simulink model "PreCondition"  (R2018b)
settings: Solver=FixedStepDiscrete  StartTime=0.0  StopTime=10.0  FixedStep=0.01  RelTol=1e-3
undefined symbols (not defined in the file or in its folder): EnergyMgLdShdRq1, HMI_2L_StMd10_Config_Val, HMI_2L_StMd11_Config_Val, HMI_2L_StMd12_Config_Val, HMI_2L_StMd13_Config_Val, HMI_2L_StMd14_Config_Val, HMI_2L_StMd15_Config_Val, HMI_2L_StMd16_Config_Val, HMI_2L_StMd17_Config_Val, HMI_2L_StMd18_Config_Val, HMI_2L_StMd19_Config_Val, HMI_2L_StMd1_Config_Val, HMI_2L_StMd20_Config_Val, HMI_2L_StMd21_Config_Val, HMI_2L_StMd22_Config_Val, HMI_2L_StMd23_Config_Val, HMI_2L_StMd24_Config_Val, HMI_2L_StMd25_Config_Val, HMI_2L_StMd26_Config_Val, HMI_2L_StMd27_Config_Val, HMI_2L_StMd28_Config_Val, HMI_2L_StMd29_Config_Val, HMI_2L_StMd2_Config_Val, HMI_2L_StMd30_Config_Val, HMI_2L_StMd31_Config_Val, HMI_2L_StMd32_Config_Val, HMI_2L_StMd3_Config_Val, HMI_2L_StMd4_Config_Val, HMI_2L_StMd5_Config_Val, HMI_2L_StMd6_Config_Val, HMI_2L_StMd7_Config_Val, HMI_2L_StMd8_Config_Val, HMI_2L_StMd9_Config_Val, HMI_2R_StMd10_Config_Val, HMI_2R_StMd11_Config_Val, HMI_2R_StMd12_Config_Val, HMI_2R_StMd13_Config_Val, HMI_2R_StMd14_Config_Val, HMI_2R_StMd15_Config_Val, HMI_2R_StMd16_Config_Val, HMI_2R_StMd17_Config_Val, HMI_2R_StMd18_Config_Val, HMI_2R_StMd19_Config_Val, HMI_2R_StMd1_Config_Val, HMI_2R_StMd20_Config_Val, HMI_2R_StMd21_Config_Val, HMI_2R_StMd22_Config_Val, HMI_2R_StMd23_Config_Val, HMI_2R_StMd24_Config_Val, HMI_2R_StMd25_Config_Val, HMI_2R_StMd26_Config_Val, HMI_2R_StMd27_Config_Val, HMI_2R_StMd28_Config_Val, HMI_2R_StMd29_Config_Val, HMI_2R_StMd2_Config_Val, HMI_2R_StMd30_Config_Val, HMI_2R_StMd31_Config_Val, HMI_2R_StMd32_Config_Val, HMI_2R_StMd3_Config_Val, HMI_2R_StMd4_Config_Val ... (+94)
(part 6 of 6)

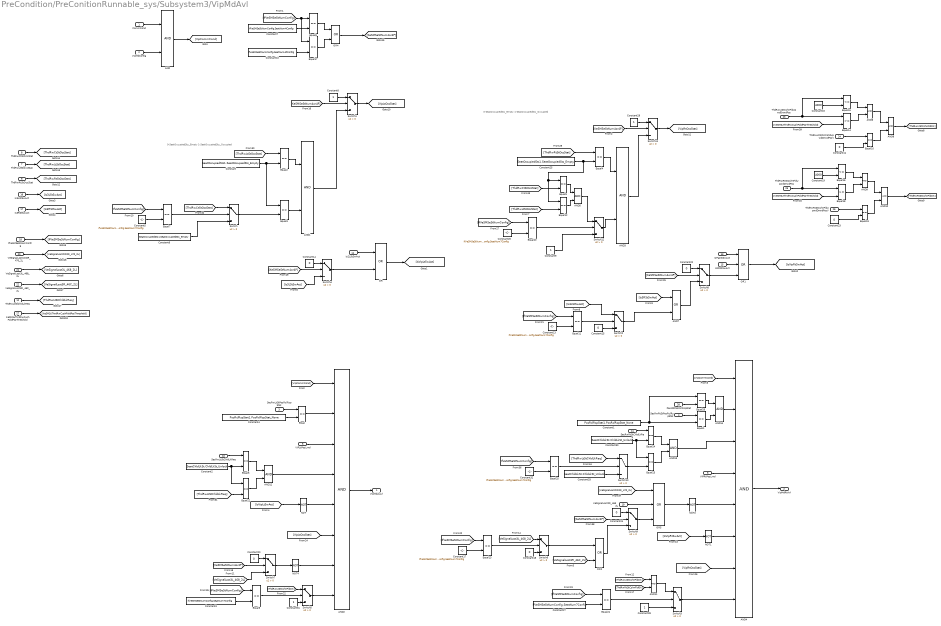
== system PreCondition/PreConitionRunnable_sys/Subsystem3/VipMdAvl ==
  note: 0-SeatOccupiedSts_Empty 1-SeatOccupiedSts_Occupied
  note: 0-SeatOccupiedSts_Empty 1-SeatOccupiedSts_Occupied
  CommCond : Inport
  VipMdConfig : Inport  Port=2
  SecRwLtStPosRclRspStat : Inport  Port=3
  SecRwRtStPosRclRspStat : Inport  Port=4
  VIPLtPosLrnd : Inport  Port=5
  VIPRtPosLrnd : Inport  Port=6
  ThdRwLtStOccStat : Inport  Port=7
  ThdRwCtStOccStat : Inport  Port=8
  ThdRwRtStOccStat : Inport  Port=9
  SecRwLtStChldLkReq : Inport  Port=10
  SecRwRtStChldLkReq : Inport  Port=11
  ThdRwLtStChldLkReq : Inport  Port=12
  IsPasStSwAct : Inport  Port=13
  Is2LStSwAct : Inport  Port=14
  Is2RStSwAct : Inport  Port=15
  Is3LStSwAct : Inport  Port=16
  Is3RStSwAct : Inport  Port=17
  IfVeSMSeStNumConfig : Inport  Port=18
  "VeSignalLost2R_463_2L " : Inport  Port=19
  VeSignalLostCODR_470_2L : Inport  Port=20
  VeSignalLost3L_468_2L : Inport  Port=21
  VeSignalLost3R_46C_2L : Inport  Port=22
  ThdRwLtStCshnFldUpwdDnwdPos : Inport  Port=23
  ThdRwLtStCshnFldUpwdDnwdPosV : Inport  Port=24
  ThdRwRtStCshnFldUpwdDnwdPos : Inport  Port=25
  ThdRwRtStCshnFldUpwdDnwdPosV : Inport  Port=26
  KeSMSuThrdRwCushFoldPosThreshold : Inport  Port=27
  PassStPosRclRspStat : Inport  Port=28
  AND{,1,3,5..6,8..14} (12 alike) : Logic  AllPortsSameDT=off  OutDataTypeStr=boolean
  AND2 : Logic  Inputs=8  AllPortsSameDT=off  OutDataTypeStr=boolean
  AND4 : Logic  Inputs=8  AllPortsSameDT=off  OutDataTypeStr=boolean
  AND7 : Logic  Operator=OR  AllPortsSameDT=off  OutDataTypeStr=boolean
  Constant : Constant  Value=SeatOccupiedSts1.SeatOccupiedSts_Empty  OutDataTypeStr=Enum:SeatOccupiedSts1
  Constant1 : Constant  Value=PosRclRspStat1.PosRclRspStat_None  OutDataTypeStr=Enum:PosRclRspStat1
  Constant10 : Constant  Value=IfVeSMSeStNumConfig.SeatNum4PConfig  OutDataTypeStr=Enum: IfVeSMSeStNumConfig
  Constant{11,14..15,20,22..24} (7 alike) : Constant  Value=0  OutDataTypeStr=boolean
  Constant13 : Constant  Value=IfVeSMSeStNumConfig.SeatNum7Config  OutDataTypeStr=Enum:IfVeSMSeStNumConfig
  Constant16 : Constant  Value=4000  OutDataTypeStr=uint16
  Constant{3,5,17,26..27,32} (6 alike) : Constant  Value=IfVeSMSeStNumConfig.SeatNum7Config  OutDataTypeStr=Enum: IfVeSMSeStNumConfig
  Constant18 : Constant  Value=0  OutDataTypeStr=uint8
  Constant19 : Constant  Value=4000  OutDataTypeStr=uint16
  Constant2 : Constant  Value=SeatChldLkSt.ChldLkSt_Unlock  OutDataTypeStr=Enum:SeatChldLkSt
  Constant25 : Constant  Value=SeatOccupiedSts1.SeatOccupiedSts_Empty  OutDataTypeStr=Enum:SeatOccupiedSts1
  Constant{8..9,28..29} (4 alike) : Constant  OutDataTypeStr=boolean
  Constant30 : Constant  Value=SeatChldLkSt.ChldLkSt_Unlock  OutDataTypeStr=Enum:SeatChldLkSt
  Constant31 : Constant  OutDataTypeStr=uint8
  Constant33 : Constant  Value=SeatChldLkSt.ChldLkSt_Unlock  OutDataTypeStr=Enum:SeatChldLkSt
  Constant4 : Constant  Value=PosRclRspStat1.PosRclRspStat_None  OutDataTypeStr=Enum:PosRclRspStat1
  Constant6 : Constant  Value=SeatOccupiedSts1.SeatOccupiedSts_Empty  OutDataTypeStr=Enum:SeatOccupiedSts1
  Constant7 : Constant  Value=IfVeSMSeStNumConfig.SeatNum4Config  OutDataTypeStr=Enum: IfVeSMSeStNumConfig
  Equal{,1..13,17,19..26} (23 alike) : RelationalOperator  Operator===  OutDataTypeStr=boolean  RndMeth=Simplest
  Equal14 : RelationalOperator  OutDataTypeStr=boolean  RndMeth=Simplest
  Equal15 : RelationalOperator  Operator=<=  OutDataTypeStr=boolean  RndMeth=Simplest
  Equal16 : RelationalOperator  Operator=<=  OutDataTypeStr=boolean  RndMeth=Simplest
  Equal18 : RelationalOperator  OutDataTypeStr=boolean  RndMeth=Simplest
  NOT{,1..2,4} (4 alike) : Logic  Operator=NOT  AllPortsSameDT=off  OutDataTypeStr=boolean
  OR : Logic  Operator=OR  AllPortsSameDT=off  OutDataTypeStr=boolean
  OR1 : Logic  Operator=OR  Inputs=3  AllPortsSameDT=off  OutDataTypeStr=boolean
  OR2 : Logic  Operator=OR  AllPortsSameDT=off  OutDataTypeStr=boolean
  OR4 : Logic  Operator=OR  AllPortsSameDT=off  OutDataTypeStr=boolean
  OR5 : Logic  Operator=OR  Inputs=3  AllPortsSameDT=off  OutDataTypeStr=boolean
  Switch{,1..12} (13 alike) : Switch  Criteria=u2 > Threshold
  VipMdLtAvl : Outport
  VipMdRtAvl : Outport  Port=2
  wires:
  CommCond/1 -> AND/1
  VipMdConfig/1 -> AND/2
  SecRwLtStPosRclRspStat/1 -> Equal/1
  Constant4/1 -> Equal/2
  Constant/1 -> Equal3/1, Equal2/2
  Equal2/1 -> AND1/1
  Equal3/1 -> AND1/2
  AND/1 -> [VipCommCond]
  Equal/1 -> AND2/2
  [VipCommCond] -> AND2/1
  SecRwLtStChldLkReq/1 -> Equal5/1
  Constant2/1 -> Equal22/1, Equal5/2
  AND2/1 -> VipMdLtAvl/1
  [VipCommCond] -> AND4/1
  AND4/1 -> VipMdRtAvl/1
  Is3LStSwAct/1 -> [Is3LStSwAct]
  Is3RStSwAct/1 -> [Is3RStSwAct]
  NOT/1 -> AND2/5
  IfVeSMSeStNumConfig/1 -> [IfVeSMSeStNumConfig]
  [IfVeSMSeStNumConfig] -> Equal7/1
  Constant5/1 -> Equal7/2
  Equal7/1 -> Switch/2
  Switch/1 -> Equal3/2
  VeSignalLost3R_46C_2L/1 -> [VeSignalLost3R_46C_2L]
  [IfVeSMSeStNumConfig] -> Equal17/1, Equal8/1
  Constant7/1 -> Equal8/2
  AND1/1 -> Switch1/3
  Constant8/1 -> Switch1/1
  [KeSMSeStNum4or4P] -> Switch4/2
  Constant14/1 -> Switch4/1
  [Is3LStSwAct] -> Switch4/3
  Switch4/1 -> OR/2
  OR/1 -> [IsVipLtSwAct]
  [IsVipLtSwAct] -> NOT/1
  [IsVipRtSwAct] -> NOT1/1
  Constant22/1 -> Switch8/1
  [KeSMSeStNum4or4P] -> Switch8/2
  [Is3RStSwAct] -> AND7/1
  AND7/1 -> Switch8/3
  OR1/1 -> [IsVipRtSwAct]
  Is2LStSwAct/1 -> OR/1
  Switch1/1 -> [VipLtOccStat]
  Switch11/1 -> [VipRtOccStat]
  [KeSMSeStNum4or4P] -> Switch11/2
  Constant29/1 -> Switch11/1
  [VipRtOccStat] -> AND4/7
  ThdRwRtStOccStat/1 -> [ThdRwRtStOccStat]
  Constant6/1 -> Switch/3
  ThdRwLtStOccStat/1 -> [ThdRwLtStOccStat]
  [ThdRwLtStOccStat] -> Equal2/1
  ThdRwCtStOccStat/1 -> [ThdRwCtStOccStat]
  [ThdRwCtStOccStat] -> Switch/1
  Constant25/1 -> Equal12/1, Equal9/1, Equal4/2
  Equal20/1 -> Switch12/2
  Equal4/1 -> AND3/1
  Switch12/1 -> AND3/2
  Constant9/1 -> Switch12/3
  Constant26/1 -> Equal20/2
  [IfVeSMSeStNumConfig] -> Equal20/1
  AND3/1 -> Switch11/3
  [ThdRwRtStOccStat] -> Equal4/1
  [ThdRwCtStOccStat] -> Equal9/2
  [ThdRwLtStOccStat] -> Equal12/2
  Equal9/1 -> AND5/1
  Equal12/1 -> AND5/2
  AND5/1 -> Switch12/1
  Constant10/1 -> Equal17/2
  Equal8/1 -> OR4/1
  Equal17/1 -> OR4/2
  OR4/1 -> [KeSMSeStNum4or4P]
  [KeSMSeStNum4or4P] -> Switch1/2
  Equal11/1 -> Switch2/2
  Constant15/1 -> Switch2/3
  Constant13/1 -> Equal11/2
  [IfVeSMSeStNumConfig] -> Equal11/1
  Switch2/1 -> AND7/2
  [Is3LStSwAct] -> Switch2/1
  VIPLtPosLrnd/1 -> AND2/3
  ThdRwLtStCshnFldUpwdDnwdPosV/1 -> Equal10/1
  Constant11/1 -> Equal10/2
  Equal15/1 -> AND6/1
  Equal14/1 -> AND6/2
  Equal10/1 -> AND8/2
  AND6/1 -> AND8/1
  AND8/1 -> [ThdRwLtStCshnFldOK]
  Equal18/1 -> AND9/2
  Equal16/1 -> AND9/1
  Constant23/1 -> Equal19/2
  ThdRwRtStCshnFldUpwdDnwdPosV/1 -> Equal19/1
  Equal19/1 -> AND10/2
  AND9/1 -> AND10/1
  AND10/1 -> [ThdRwRtStCshnFldOK]
  Constant27/1 -> Equal21/2
  [IfVeSMSeStNumConfig] -> Equal21/1
  Equal21/1 -> Switch3/2
  Constant28/1 -> Switch3/3
  NOT1/1 -> AND4/6
  Switch8/1 -> OR1/3
  Is2RStSwAct/1 -> OR1/2
  IsPasStSwAct/1 -> OR1/1
  VeSignalLostCODR_470_2L/1 -> [VeSignalLostCODR_470_2L]
  SecRwRtStPosRclRspStat/1 -> Equal1/1
  Constant1/1 -> Equal26/1, Equal1/2
  ThdRwLtStChldLkReq/1 -> [ThdRwLtStChldLkReq]
  [ThdRwLtStChldLkReq] -> Equal22/2
  Equal5/1 -> AND12/1
  Equal22/1 -> AND12/2
  AND12/1 -> AND2/4
  Equal23/1 -> AND13/2
  Equal24/1 -> AND13/1
  Constant30/1 -> Equal24/2, Equal23/1
  VIPRtPosLrnd/1 -> AND4/4
  SecRwRtStChldLkReq/1 -> Equal24/1
  AND13/1 -> AND4/3
  ThdRwLtStCshnFldUpwdDnwdPos/1 -> Equal15/1, Equal14/1
  Constant16/1 -> Equal15/2
  ThdRwRtStCshnFldUpwdDnwdPos/1 -> Equal16/1, Equal18/1
  Constant19/1 -> Equal16/2
  Constant3/1 -> Equal6/2
  Equal6/1 -> Switch5/2
  Constant31/1 -> Switch5/3
  [IfVeSMSeStNumConfig] -> Equal6/1
  [ThdRwLtStCshnFldOK] -> Switch5/1
  Equal25/1 -> Switch10/2
  Constant32/1 -> Equal25/2
  [ThdRwLtStChldLkReq] -> Switch10/1
  [IfVeSMSeStNumConfig] -> Equal25/1
  Constant33/1 -> Switch10/3
  Switch10/1 -> Equal23/2
  [VipLtOccStat] -> AND2/6
  Switch5/1 -> AND2/8
  [VeSignalLost3L_468_2L] -> Switch7/3
  Switch7/1 -> NOT4/1
  NOT4/1 -> AND2/7
  [KeSMSeStNum4or4P] -> Switch7/2
  Constant20/1 -> Switch7/1
  VeSignalLost3L_468_2L/1 -> [VeSignalLost3L_468_2L]
  [VeSignalLostCODR_470_2L] -> OR5/1
  Switch9/1 -> OR5/3
  [KeSMSeStNum4or4P] -> Switch9/2
  Constant24/1 -> Switch9/1
  [IfVeSMSeStNumConfig] -> Equal13/1
  Constant18/1 -> Switch6/3
  Switch6/1 -> OR2/1
  [VeSignalLost3R_46C_2L] -> OR2/2
  Equal13/1 -> Switch6/2
  [VeSignalLost3L_468_2L] -> Switch6/1
  "VeSignalLost2R_463_2L "/1 -> OR5/2
  OR2/1 -> Switch9/3
  Constant17/1 -> Equal13/2
  OR5/1 -> NOT2/1
  NOT2/1 -> AND4/5
  AND11/1 -> Switch3/1
  [ThdRwRtStCshnFldOK] -> AND11/2
  [ThdRwLtStCshnFldOK] -> AND11/1
  Switch3/1 -> AND4/8
  KeSMSuThrdRwCushFoldPosThreshold/1 -> [KeSMSuThrdRwCushFoldPosThreshold]
  [KeSMSuThrdRwCushFoldPosThreshold] -> Equal14/2
  [KeSMSuThrdRwCushFoldPosThreshold] -> Equal18/2
  PassStPosRclRspStat/1 -> Equal26/2
  Equal26/1 -> AND14/1
  Equal1/1 -> AND14/2
  AND14/1 -> AND4/2

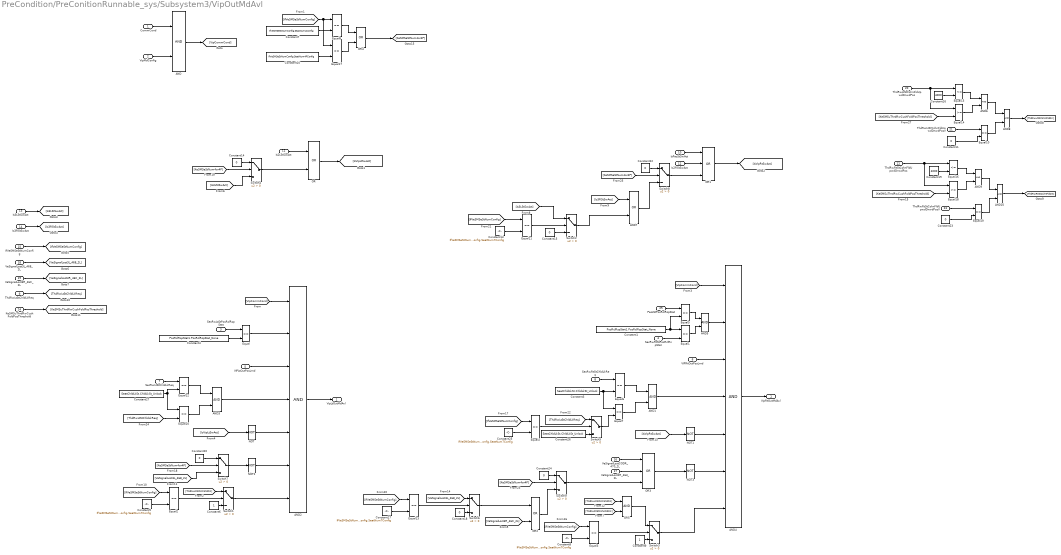
== system PreCondition/PreConitionRunnable_sys/Subsystem3/VipOutMdAvl ==
  CommCond : Inport
  VipMdConfig : Inport  Port=2
  SecRwLtStPosRclRspStat : Inport  Port=3
  SecRwRtStPosRclRspStat : Inport  Port=4
  VIPLtOutPosLrnd : Inport  Port=5
  VIPRtOutPosLrnd : Inport  Port=6
  SecRwLtStChldLkReq : Inport  Port=7
  SecRwRtStChldLkReq : Inport  Port=8
  ThdRwLtStChldLkReq : Inport  Port=9
  IsPasStSwAct : Inport  Port=10
  Is2LStSwAct : Inport  Port=11
  Is2RStSwAct : Inport  Port=12
  Is3LStSwAct : Inport  Port=13
  Is3RStSwAct : Inport  Port=14
  IfVeSMSeStNumConfig : Inport  Port=15
  VeSignalLostCODR_470_2L : Inport  Port=16
  VeSignalLost2R_463_2L : Inport  Port=17
  VeSignalLost3L_468_2L : Inport  Port=18
  VeSignalLost3R_46C_2L : Inport  Port=19
  ThdRwLtStCshnFldUpwdDnwdPos : Inport  Port=20
  ThdRwLtStCshnFldUpwdDnwdPosV : Inport  Port=21
  ThdRwRtStCshnFldUpwdDnwdPos : Inport  Port=22
  ThdRwRtStCshnFldUpwdDnwdPosV : Inport  Port=23
  KeSMSuThrdRwCushFoldPosThreshold : Inport  Port=24
  PassStPosRclRspStat : Inport  Port=25
  AND{,1,3,5..6,8..10} (8 alike) : Logic  AllPortsSameDT=off  OutDataTypeStr=boolean
  AND2 : Logic  Inputs=7  AllPortsSameDT=off  OutDataTypeStr=boolean
  AND4 : Logic  Inputs=7  AllPortsSameDT=off  OutDataTypeStr=boolean
  AND7 : Logic  Operator=OR  AllPortsSameDT=off  OutDataTypeStr=boolean
  Constant1 : Constant  Value=PosRclRspStat1.PosRclRspStat_None  OutDataTypeStr=Enum:PosRclRspStat1
  Constant10 : Constant  Value=IfVeSMSeStNumConfig.SeatNum4PConfig  OutDataTypeStr=Enum: IfVeSMSeStNumConfig
  Constant{11,14..15,20,22..24} (7 alike) : Constant  Value=0  OutDataTypeStr=boolean
  Constant13 : Constant  Value=IfVeSMSeStNumConfig.SeatNum7Config  OutDataTypeStr=Enum:IfVeSMSeStNumConfig
  Constant16 : Constant  Value=4000  OutDataTypeStr=uint16
  Constant{5,8,17,25} (4 alike) : Constant  Value=IfVeSMSeStNumConfig.SeatNum7Config  OutDataTypeStr=Enum: IfVeSMSeStNumConfig
  Constant18 : Constant  Value=0  OutDataTypeStr=uint8
  Constant19 : Constant  Value=4000  OutDataTypeStr=uint16
  Constant26 : Constant  Value=SeatChldLkSt.ChldLkSt_Unlock  OutDataTypeStr=Enum:SeatChldLkSt
  Constant27 : Constant  Value=SeatChldLkSt.ChldLkSt_Unlock  OutDataTypeStr=Enum:SeatChldLkSt
  Constant3 : Constant  Value=SeatChldLkSt.ChldLkSt_Unlock  OutDataTypeStr=Enum:SeatChldLkSt
  Constant4 : Constant  Value=PosRclRspStat1.PosRclRspStat_None  OutDataTypeStr=Enum:PosRclRspStat1
  Constant6 : Constant  OutDataTypeStr=uint8
  Constant7 : Constant  Value=IfVeSMSeStNumConfig.SeatNum4Config  OutDataTypeStr=Enum: IfVeSMSeStNumConfig
  Constant9 : Constant  OutDataTypeStr=uint8
  Equal{,1..8,10..13,17,19..20} (16 alike) : RelationalOperator  Operator===  OutDataTypeStr=boolean  RndMeth=Simplest
  Equal14 : RelationalOperator  OutDataTypeStr=boolean  RndMeth=Simplest
  Equal15 : RelationalOperator  Operator=<=  OutDataTypeStr=boolean  RndMeth=Simplest
  Equal16 : RelationalOperator  Operator=<=  OutDataTypeStr=boolean  RndMeth=Simplest
  Equal18 : RelationalOperator  OutDataTypeStr=boolean  RndMeth=Simplest
  NOT{,1..3} (4 alike) : Logic  Operator=NOT  AllPortsSameDT=off  OutDataTypeStr=boolean
  OR : Logic  Operator=OR  AllPortsSameDT=off  OutDataTypeStr=boolean
  OR1 : Logic  Operator=OR  Inputs=3  AllPortsSameDT=off  OutDataTypeStr=boolean
  OR2 : Logic  Operator=OR  AllPortsSameDT=off  OutDataTypeStr=boolean
  OR3 : Logic  Operator=OR  Inputs=3  AllPortsSameDT=off  OutDataTypeStr=boolean
  OR4 : Logic  Operator=OR  AllPortsSameDT=off  OutDataTypeStr=boolean
  OR5 : Logic  AllPortsSameDT=off  OutDataTypeStr=boolean
  Switch{1..9} (9 alike) : Switch  Criteria=u2 > Threshold
  VipLtOutMdAvl : Outport
  VipRtOutMdAvl : Outport  Port=2
  wires:
  VIPRtOutPosLrnd/1 -> AND4/3
  VIPLtOutPosLrnd/1 -> AND2/3
  [Is3LStSwAct] -> Switch2/1
  Switch2/1 -> AND7/2
  [IfVeSMSeStNumConfig] -> Equal11/1
  Constant13/1 -> Equal11/2
  Constant15/1 -> Switch2/3
  Equal11/1 -> Switch2/2
  OR4/1 -> [KeSMSeStNum4or4P]
  Equal17/1 -> OR4/2
  Equal8/1 -> OR4/1
  Constant10/1 -> Equal17/2
  Is2LStSwAct/1 -> OR/1
  OR3/1 -> NOT3/1
  OR1/1 -> [IsVipRtSwAct]
  AND7/1 -> Switch8/3
  [Is3RStSwAct] -> AND7/1
  [KeSMSeStNum4or4P] -> Switch8/2
  Constant22/1 -> Switch8/1
  [IsVipRtSwAct] -> NOT1/1
  [IsVipLtSwAct] -> NOT/1
  OR/1 -> [IsVipLtSwAct]
  Switch4/1 -> OR/2
  [Is3LStSwAct] -> Switch4/3
  Constant14/1 -> Switch4/1
  [KeSMSeStNum4or4P] -> Switch4/2
  Constant7/1 -> Equal8/2
  [IfVeSMSeStNumConfig] -> Equal8/1, Equal17/1
  NOT3/1 -> AND4/6
  NOT2/1 -> AND2/6
  VeSignalLost3R_46C_2L/1 -> [VeSignalLost3R_46C_2L]
  IfVeSMSeStNumConfig/1 -> [IfVeSMSeStNumConfig]
  NOT1/1 -> AND4/5
  NOT/1 -> AND2/5
  Is3RStSwAct/1 -> [Is3RStSwAct]
  Is3LStSwAct/1 -> [Is3LStSwAct]
  AND4/1 -> VipRtOutMdAvl/1
  SecRwRtStChldLkReq/1 -> Equal6/1
  Constant3/1 -> Equal7/1, Equal6/2
  [VipCommCond] -> AND4/1
  AND2/1 -> VipLtOutMdAvl/1
  [VipCommCond] -> AND2/1
  Equal/1 -> AND2/2
  AND/1 -> [VipCommCond]
  Constant1/1 -> Equal5/2, Equal1/1
  SecRwRtStPosRclRspStat/1 -> Equal1/2
  Constant4/1 -> Equal/2
  SecRwLtStPosRclRspStat/1 -> Equal/1
  VipMdConfig/1 -> AND/2
  CommCond/1 -> AND/1
  Switch8/1 -> OR1/3
  Is2RStSwAct/1 -> OR1/2
  IsPasStSwAct/1 -> OR1/1
  VeSignalLost2R_463_2L/1 -> OR3/2
  VeSignalLostCODR_470_2L/1 -> OR3/1
  AND6/1 -> AND8/1
  Equal14/1 -> AND6/2
  Equal15/1 -> AND6/1
  ThdRwLtStCshnFldUpwdDnwdPosV/1 -> Equal10/1
  Constant11/1 -> Equal10/2
  [KeSMSuThrdRwCushFoldPosThreshold] -> Equal18/2
  ThdRwRtStCshnFldUpwdDnwdPosV/1 -> Equal19/1
  Equal19/1 -> AND10/2
  Equal16/1 -> AND9/1
  Equal10/1 -> AND8/2
  Equal18/1 -> AND9/2
  AND8/1 -> [ThdRwLtStCshnFldOK]
  Constant23/1 -> Equal19/2
  AND9/1 -> AND10/1
  AND10/1 -> [ThdRwRtStCshnFldOK]
  Switch1/1 -> AND2/7
  [IfVeSMSeStNumConfig] -> Equal2/1
  Constant5/1 -> Equal2/2
  Constant6/1 -> Switch1/3
  Equal2/1 -> Switch1/2
  [ThdRwLtStCshnFldOK] -> Switch1/1
  Constant8/1 -> Equal3/2
  Equal3/1 -> Switch3/2
  Constant9/1 -> Switch3/3
  [IfVeSMSeStNumConfig] -> Equal3/1
  [ThdRwLtStCshnFldOK] -> OR5/1
  [ThdRwRtStCshnFldOK] -> OR5/2
  OR5/1 -> Switch3/1
  Switch3/1 -> AND4/7
  Equal4/1 -> Switch5/2
  Constant25/1 -> Equal4/2
  [IfVeSMSeStNumConfig] -> Equal4/1
  Switch5/1 -> Equal7/2
  Constant26/1 -> Switch5/3
  Equal6/1 -> AND1/1
  Equal7/1 -> AND1/2
  AND1/1 -> AND4/4
  ThdRwLtStChldLkReq/1 -> [ThdRwLtStChldLkReq]
  [ThdRwLtStChldLkReq] -> Switch5/1
  Equal20/1 -> AND3/2
  Equal12/1 -> AND3/1
  Constant27/1 -> Equal12/2, Equal20/1
  SecRwLtStChldLkReq/1 -> Equal12/1
  AND3/1 -> AND2/4
  [ThdRwLtStChldLkReq] -> Equal20/2
  Constant16/1 -> Equal15/2
  ThdRwLtStCshnFldUpwdDnwdPos/1 -> Equal14/1, Equal15/1
  Constant19/1 -> Equal16/2
  ThdRwRtStCshnFldUpwdDnwdPos/1 -> Equal18/1, Equal16/1
  Constant20/1 -> Switch7/1
  [KeSMSeStNum4or4P] -> Switch7/2
  [VeSignalLost3L_468_2L] -> Switch7/3
  Switch7/1 -> NOT2/1
  VeSignalLost3L_468_2L/1 -> [VeSignalLost3L_468_2L]
  [IfVeSMSeStNumConfig] -> Equal13/1
  Constant24/1 -> Switch9/1
  Switch9/1 -> OR3/3
  [VeSignalLost3R_46C_2L] -> OR2/2
  Equal13/1 -> Switch6/2
  Constant17/1 -> Equal13/2
  Switch6/1 -> OR2/1
  Constant18/1 -> Switch6/3
  [KeSMSeStNum4or4P] -> Switch9/2
  [VeSignalLost3L_468_2L] -> Switch6/1
  OR2/1 -> Switch9/3
  KeSMSuThrdRwCushFoldPosThreshold/1 -> [KeSMSuThrdRwCushFoldPosThreshold]
  [KeSMSuThrdRwCushFoldPosThreshold] -> Equal14/2
  PassStPosRclRspStat/1 -> Equal5/1
  Equal5/1 -> AND5/1
  Equal1/1 -> AND5/2
  AND5/1 -> AND4/2

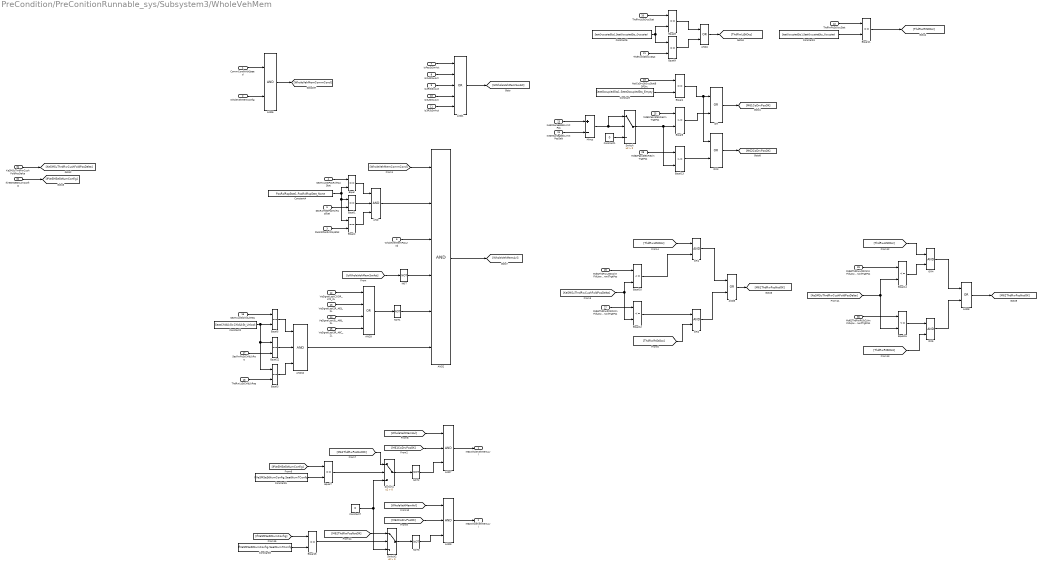
== system PreCondition/PreConitionRunnable_sys/Subsystem3/WholeVehMem ==
  CommCondWithSpeed : Inport
  WholeVehMemConfig : Inport  Port=2
  PassStPosRclRspStat : Inport  Port=3
  SecRwLtStPosRclRspStat : Inport  Port=4
  SecRwRtStPosRclRspStat : Inport  Port=5
  WholeVehMemPosLrnd : Inport  Port=6
  IsPasStSwAct : Inport  Port=7
  Is2LStSwAct : Inport  Port=8
  Is2RStSwAct : Inport  Port=9
  Is3LStSwAct : Inport  Port=10
  Is3RStSwAct : Inport  Port=11
  VeSignalLostCODR_470_2L : Inport  Port=12
  VeSignalLost2R_463_2L : Inport  Port=13
  VeSignalLost3L_468_2L : Inport  Port=14
  VeSignalLost3R_46C_2L : Inport  Port=15
  SecRwLtStChldLkReq : Inport  Port=16
  SecRwRtStChldLkReq : Inport  Port=17
  ThdRwLtStChldLkReq : Inport  Port=18
  NotCoDrvStOccStatBDFSrc : Inport  Port=19
  ThdRwLtStOccStat : Inport  Port=20
  ThdRwCtStOccStat : Inport  Port=21
  ThdRwRtStOccStat : Inport  Port=22
  KeSMSwSeatBkLimitPos : Inport  Port=23
  KeSMSwSeatBkLimitPosDelt : Inport  Port=24
  Md61PassStBkReclnTrgtPos : Inport  Port=25
  Md61ThdRwLtStCshnFldUpwdDnwdTrgtPos : Inport  Port=26
  Md61ThdRwRtStCshnFldUpwdDnwdTrgtPos : Inport  Port=27
  Md62PassStBkReclnTrgtPos : Inport  Port=28
  Md62ThdRwLtStCshnFldUpwdDnwdTrgtPos : Inport  Port=29
  Md62ThdRwRtStCshnFldUpwdDnwdTrgtPos : Inport  Port=30
  KeSMSuThrdRwCushFoldPosDelta : Inport  Port=31
  IfVeSMSeStNumConfig : Inport  Port=32
  AND{,7,9,12} (4 alike) : Logic  Inputs=3  AllPortsSameDT=off  OutDataTypeStr=boolean
  AND1 : Logic  Operator=OR  Inputs=5  AllPortsSameDT=off  OutDataTypeStr=boolean
  AND2 : Logic  Inputs=6  AllPortsSameDT=off  OutDataTypeStr=boolean
  AND3 : Logic  Operator=OR  Inputs=4  AllPortsSameDT=off  OutDataTypeStr=boolean
  AND4 : Logic  Operator=OR  AllPortsSameDT=off  OutDataTypeStr=boolean
  AND5 : Logic  Operator=OR  AllPortsSameDT=off  OutDataTypeStr=boolean
  AND6 : Logic  AllPortsSameDT=off  OutDataTypeStr=boolean
  AND8 : Logic  Operator=OR  AllPortsSameDT=off  OutDataTypeStr=boolean
  Constant : Constant  Value=SeatOccupiedSts1.SeatOccupiedSts_Empty  OutDataTypeStr=Enum:SeatOccupiedSts1
  Constant1 : Constant  Value=0  OutDataTypeStr=uint16
  Constant2 : Constant  Value=SeatChldLkSt.ChldLkSt_Unlock  OutDataTypeStr=Enum:SeatChldLkSt
  Constant3 : Constant  Value=SeatOccupiedSts1.SeatOccupiedSts_Occupied  OutDataTypeStr=Enum:SeatOccupiedSts1
  Constant4 : Constant  Value=PosRclRspStat1.PosRclRspStat_None  OutDataTypeStr=Enum:PosRclRspStat1
  Constant5 : Constant  Value=IfVeSMSeStNumConfig.SeatNum7Config  OutDataTypeStr=Enum:IfVeSMSeStNumConfig
  Constant6 : Constant  Value=SeatOccupiedSts1.SeatOccupiedSts_Occupied  OutDataTypeStr=Enum:SeatOccupiedSts1
  Constant7 : Constant  Value=0  OutDataTypeStr=uint8
  Constant8 : Constant  Value=IfVeSMSeStNumConfig.SeatNum7Config  OutDataTypeStr=Enum:IfVeSMSeStNumConfig
  Equal{,1..5,7..9,11,16,22} (12 alike) : RelationalOperator  Operator===  OutDataTypeStr=boolean  RndMeth=Simplest
  Equal{10,12,14..15} (4 alike) : RelationalOperator  Operator=<=  OutDataTypeStr=boolean  RndMeth=Simplest
  Equal13 : RelationalOperator  OutDataTypeStr=boolean  RndMeth=Simplest
  Equal6 : RelationalOperator  OutDataTypeStr=boolean  RndMeth=Simplest
  Minus : Sum  Inputs=+-
  NOT{,1..3} (4 alike) : Logic  Operator=NOT  AllPortsSameDT=off  OutDataTypeStr=boolean
  OR : Logic  Operator=OR  AllPortsSameDT=off  OutDataTypeStr=boolean
  OR{1..2,4..5} (4 alike) : Logic  AllPortsSameDT=off  OutDataTypeStr=boolean
  OR3 : Logic  Operator=OR  AllPortsSameDT=off  OutDataTypeStr=boolean
  Switch : Switch  Criteria=u2 > Threshold
  Switch1 : Switch  Criteria=u2 > Threshold
  Switch2 : Switch  Criteria=u2 > Threshold
  M61WholeVehMemAvl : Outport
  M62WholeVehMemAvl : Outport  Port=2
  wires:
  WholeVehMemConfig/1 -> AND6/2
  AND6/1 -> [WholeVehMemCommCond]
  CommCondWithSpeed/1 -> AND6/1
  [WholeVehMemCommCond] -> AND2/1
  Equal22/1 -> AND12/2
  SecRwLtStChldLkReq/1 -> Equal5/1
  SecRwLtStPosRclRspStat/1 -> Equal/1
  Constant2/1 -> Equal3/1, Equal22/1, Equal5/2
  Constant4/1 -> Equal/2, Equal2/1, Equal1/1
  WholeVehMemPosLrnd/1 -> AND2/3
  Equal5/1 -> AND12/1
  SecRwRtStPosRclRspStat/1 -> Equal1/2
  PassStPosRclRspStat/1 -> Equal2/2
  Equal1/1 -> AND/2
  Equal/1 -> AND/1
  Equal2/1 -> AND/3
  AND/1 -> AND2/2
  AND1/1 -> [IsWholeVehMemSwAct]
  IsPasStSwAct/1 -> AND1/1
  Is2LStSwAct/1 -> AND1/2
  Is2RStSwAct/1 -> AND1/3
  [IsWholeVehMemSwAct] -> NOT/1
  NOT/1 -> AND2/4
  VeSignalLost3L_468_2L/1 -> AND3/3
  VeSignalLostCODR_470_2L/1 -> AND3/1
  VeSignalLost3R_46C_2L/1 -> AND3/4
  VeSignalLost2R_463_2L/1 -> AND3/2
  AND3/1 -> NOT1/1
  NOT1/1 -> AND2/5
  ThdRwLtStChldLkReq/1 -> Equal3/2
  SecRwRtStChldLkReq/1 -> Equal22/2
  Equal3/1 -> AND12/3
  AND12/1 -> AND2/6
  Constant/1 -> Equal4/2
  NotCoDrvStOccStatBDFSrc/1 -> Equal4/1
  KeSMSwSeatBkLimitPos/1 -> Minus/1
  KeSMSwSeatBkLimitPosDelt/1 -> Minus/2
  Minus/1 -> Switch/1, Switch/2
  Constant1/1 -> Switch/3
  Switch/1 -> Equal6/2, Equal13/2
  Md61PassStBkReclnTrgtPos/1 -> Equal6/1
  Equal4/1 -> OR3/1, OR/1
  Equal6/1 -> OR/2
  OR/1 -> [M61CoDrvPosOK]
  KeSMSuThrdRwCushFoldPosDelta/1 -> [KeSMSuThrdRwCushFoldPosDelta]
  Constant5/1 -> Equal7/2
  [IfVeSMSeStNumConfig] -> Equal7/1
  Constant6/1 -> Equal9/1, Equal8/2
  IfVeSMSeStNumConfig/1 -> [IfVeSMSeStNumConfig]
  ThdRwLtStOccStat/1 -> Equal8/1
  ThdRwCtStOccStat/1 -> Equal9/2
  Md61ThdRwLtStCshnFldUpwdDnwdTrgtPos/1 -> Equal10/1
  [KeSMSuThrdRwCushFoldPosDelta] -> Equal10/2, Equal12/2
  Equal8/1 -> AND4/1
  Equal9/1 -> AND4/2
  Equal10/1 -> OR1/2
  AND4/1 -> [ThdRwLtStOcc]
  Constant3/1 -> Equal11/2
  ThdRwRtStOccStat/1 -> Equal11/1
  Equal11/1 -> [ThdRwRtStOcc]
  [ThdRwLtStOcc] -> OR1/1
  Md61ThdRwRtStCshnFldUpwdDnwdTrgtPos/1 -> Equal12/1
  [ThdRwRtStOcc] -> OR2/2
  Equal12/1 -> OR2/1
  OR1/1 -> AND5/1
  OR2/1 -> AND5/2
  AND5/1 -> [M61ThdRwPosNotOK]
  Equal7/1 -> Switch1/2
  [M61ThdRwPosNotOK] -> Switch1/1
  Switch1/1 -> NOT2/1
  Constant7/1 -> Switch1/3, Switch2/3
  AND2/1 -> [WholeVehMemAvl]
  AND7/1 -> M61WholeVehMemAvl/1
  NOT2/1 -> AND7/3
  [M61CoDrvPosOK] -> AND7/2
  [WholeVehMemAvl] -> AND7/1
  Md62PassStBkReclnTrgtPos/1 -> Equal13/1
  Equal13/1 -> OR3/2
  OR3/1 -> [M62CoDrvPosOK]
  Md62ThdRwLtStCshnFldUpwdDnwdTrgtPos/1 -> Equal14/1
  Md62ThdRwRtStCshnFldUpwdDnwdTrgtPos/1 -> Equal15/1
  [KeSMSuThrdRwCushFoldPosDelta] -> Equal15/2, Equal14/2
  [ThdRwLtStOcc] -> OR4/1
  Equal14/1 -> OR4/2
  Equal15/1 -> OR5/1
  [ThdRwRtStOcc] -> OR5/2
  OR4/1 -> AND8/1
  OR5/1 -> AND8/2
  AND8/1 -> [M62ThdRwPosNotOK]
  [M62ThdRwPosNotOK] -> Switch2/1
  Equal16/1 -> Switch2/2
  [IfVeSMSeStNumConfig] -> Equal16/1
  Constant8/1 -> Equal16/2
  [WholeVehMemAvl] -> AND9/1
  [M62CoDrvPosOK] -> AND9/2
  Switch2/1 -> NOT3/1
  NOT3/1 -> AND9/3
  AND9/1 -> M62WholeVehMemAvl/1
  Is3LStSwAct/1 -> AND1/4
  Is3RStSwAct/1 -> AND1/5

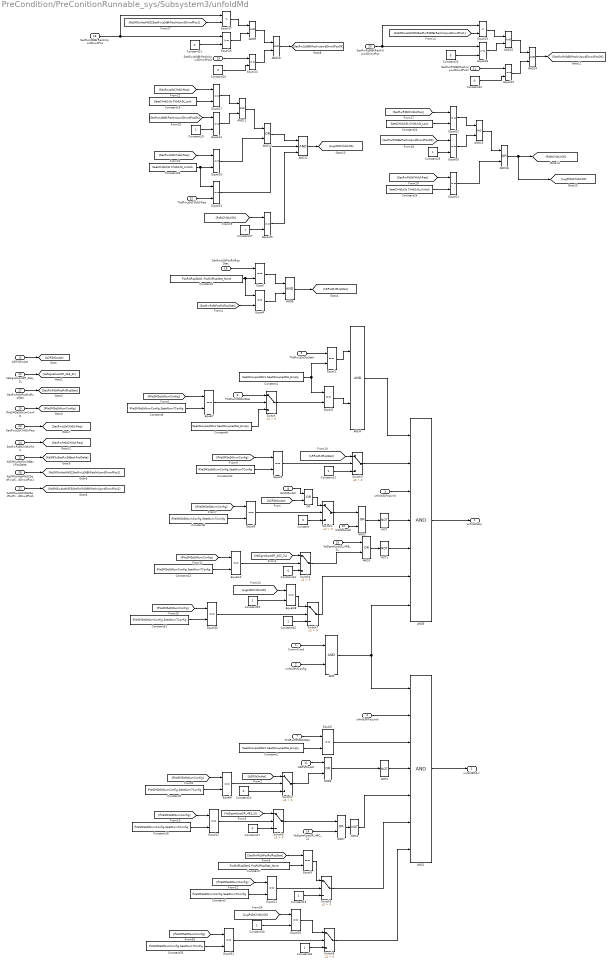
== system PreCondition/PreConitionRunnable_sys/Subsystem3/unfoldMd ==
  CommCond : Inport
  unfoldMdConfig : Inport  Port=2
  unfold3LPosLrnd : Inport  Port=3
  unfold3RPosLrnd : Inport  Port=4
  ThdRwLtStOccStat : Inport  Port=5
  ThdRwCtStOccStat : Inport  Port=6
  ThdRwRtStOccStat : Inport  Port=7
  Is2LStSwAct : Inport  Port=8
  Is2RStSwAct : Inport  Port=9
  Is3LStSwAct : Inport  Port=10
  Is3RStSwAct : Inport  Port=11
  VeSignalLost2R_463_2L : Inport  Port=12
  VeSignalLost3L_468_2L : Inport  Port=13
  VeSignalLost3R_46C_2L : Inport  Port=14
  IfVeSMSeStNumConfig : Inport  Port=15
  SecRwLtStPosRclRspStat : Inport  Port=16
  SecRwRtStPosRclRspStat : Inport  Port=17
  SecRwLtStBkReclnUpwdDnwdPos : Inport  Port=18
  SecRwLtStBkReclnUpwdDnwdPosV : Inport  Port=19
  SecRwRtStBkReclnUpwdDnwdPos : Inport  Port=20
  SecRwRtStBkReclnUpwdDnwdPosV : Inport  Port=21
  ThdRwLtStChldLkReq : Inport  Port=22
  SecRwLtStChldLkReq : Inport  Port=23
  SecRwRtStChldLkReq : Inport  Port=24
  KeSMSuSecRwStBackPosDelta : Inport  Port=25
  KeSMSwAcsMd32SecRwLtStBkReclnUpwdDnwdPos1 : Inport  Port=26
  KeSMSwAcsMd53SecRwRtStBkReclnUpwdDnwdPos1 : Inport  Port=27
  AND{,4,8..11,14..16} (9 alike) : Logic  AllPortsSameDT=off  OutDataTypeStr=boolean
  AND1 : Logic  Inputs=7  AllPortsSameDT=off  OutDataTypeStr=boolean
  AND12 : Logic  Inputs=3  AllPortsSameDT=off  OutDataTypeStr=boolean
  AND{2..3,6..7,13,18} (6 alike) : Logic  Operator=OR  AllPortsSameDT=off  OutDataTypeStr=boolean
  AND5 : Logic  Inputs=7  AllPortsSameDT=off  OutDataTypeStr=boolean
  Constant{,10,14,17} (4 alike) : Constant  Value=0  OutDataTypeStr=uint8
  Constant1 : Constant  Value=SeatOccupiedSts1.SeatOccupiedSts_Empty  OutDataTypeStr=Enum:SeatOccupiedSts1
  Constant{3,5,8..9,11,13,16,31,33} (9 alike) : Constant  Value=IfVeSMSeStNumConfig.SeatNum7Config  OutDataTypeStr=Enum:IfVeSMSeStNumConfig
  Constant{12,15,32,34} (4 alike) : Constant  OutDataTypeStr=uint8
  Constant18 : Constant  Value=SeatChldLkSt.ChldLkSt_Lock  OutDataTypeStr=Enum:SeatChldLkSt
  Constant{19,25,27,29..30} (5 alike) : Constant  OutDataTypeStr=boolean
  Constant2 : Constant  Value=SeatOccupiedSts1.SeatOccupiedSts_Empty  OutDataTypeStr=Enum:SeatOccupiedSts1
  Constant20 : Constant  Value=0  OutDataTypeStr=boolean
  Constant21 : Constant  Value=0  OutDataTypeStr=uint16
  Constant22 : Constant  Value=0  OutDataTypeStr=boolean
  Constant23 : Constant  Value=0  OutDataTypeStr=uint16
  Constant24 : Constant  Value=SeatChldLkSt.ChldLkSt_Lock  OutDataTypeStr=Enum:SeatChldLkSt
  Constant26 : Constant  Value=SeatChldLkSt.ChldLkSt_Unlock  OutDataTypeStr=Enum:SeatChldLkSt
  Constant28 : Constant  Value=SeatChldLkSt.ChldLkSt_Unlock  OutDataTypeStr=Enum:SeatChldLkSt
  Constant4 : Constant  Value=PosRclRspStat1.PosRclRspStat_None  OutDataTypeStr=Enum:PosRclRspStat1
  Constant6 : Constant  Value=SeatOccupiedSts1.SeatOccupiedSts_Empty  OutDataTypeStr=Enum:SeatOccupiedSts1
  Constant7 : Constant  Value=PosRclRspStat1.PosRclRspStat_None  OutDataTypeStr=Enum:PosRclRspStat1
  Equal{,1..15,20..23,25..31} (27 alike) : RelationalOperator  Operator===  OutDataTypeStr=boolean  RndMeth=Simplest
  Equal16 : RelationalOperator  OutDataTypeStr=boolean  RndMeth=Simplest
  Equal17 : RelationalOperator  Operator=<  OutDataTypeStr=boolean  RndMeth=Simplest
  Equal18 : RelationalOperator  OutDataTypeStr=boolean  RndMeth=Simplest
  Equal19 : RelationalOperator  Operator=<  OutDataTypeStr=boolean  RndMeth=Simplest
  NOT{,1..3} (4 alike) : Logic  Operator=NOT  AllPortsSameDT=off  OutDataTypeStr=boolean
  OR : Logic  Operator=OR  AllPortsSameDT=off  OutDataTypeStr=boolean
  Switch{,1..8} (9 alike) : Switch  Criteria=u2 > Threshold
  "unfold3LAvl " : Outport
  "unfold3RAvl " : Outport  Port=2
  wires:
  AND5/1 -> "unfold3LAvl "/1
  Constant6/1 -> Switch/3
  Constant5/1 -> Equal7/2
  Constant1/1 -> Equal1/2, Equal3/1
  Equal7/1 -> Switch/2
  Equal3/1 -> AND4/2
  Switch/1 -> Equal3/2
  Equal1/1 -> AND4/1
  ThdRwLtStOccStat/1 -> Equal1/1
  ThdRwCtStOccStat/1 -> Switch/1
  ThdRwRtStOccStat/1 -> Equal2/1
  Constant2/1 -> Equal2/2
  AND1/1 -> "unfold3RAvl "/1
  CommCond/1 -> AND/1
  unfoldMdConfig/1 -> AND/2
  AND/1 -> AND5/7, AND1/1
  unfold3RPosLrnd/1 -> AND1/2
  Equal2/1 -> AND1/3
  NOT2/1 -> AND1/4
  NOT3/1 -> AND1/5
  AND2/1 -> NOT/1
  Is2RStSwAct/1 -> [Is2RStSwAct]
  VeSignalLost2R_463_2L/1 -> [VeSignalLost2R_463_2L]
  AND3/1 -> NOT1/1
  AND6/1 -> NOT2/1
  Is3RStSwAct/1 -> AND6/1
  AND7/1 -> NOT3/1
  Constant4/1 -> Equal4/1, Equal/2
  SecRwLtStPosRclRspStat/1 -> Equal/1
  Equal/1 -> AND8/1
  Equal4/1 -> AND8/2
  NOT1/1 -> AND5/5
  NOT/1 -> AND5/4
  unfold3LPosLrnd/1 -> AND5/3
  AND4/1 -> AND5/1
  Constant7/1 -> Equal5/2
  SecRwRtStPosRclRspStat/1 -> [SecRwRtStPosRclRspStat]
  [SecRwRtStPosRclRspStat] -> Equal5/1
  Constant8/1 -> Equal6/2
  Equal6/1 -> Switch1/2
  IfVeSMSeStNumConfig/1 -> [IfVeSMSeStNumConfig]
  [IfVeSMSeStNumConfig] -> Equal7/1
  [IfVeSMSeStNumConfig] -> Equal6/1
  Is2LStSwAct/1 -> OR/1
  [Is2RStSwAct] -> OR/2
  OR/1 -> Switch1/1
  Constant/1 -> Switch1/3
  Switch1/1 -> AND2/1
  Is3LStSwAct/1 -> AND2/2
  [IfVeSMSeStNumConfig] -> Equal8/1
  Constant9/1 -> Equal8/2
  Constant10/1 -> Switch2/3
  Equal8/1 -> Switch2/2
  [Is2RStSwAct] -> Switch2/1
  Switch2/1 -> AND6/2
  AND8/1 -> [LRPosRclRspStat]
  [IfVeSMSeStNumConfig] -> Equal9/1
  Constant11/1 -> Equal9/2
  Equal9/1 -> Switch3/2
  [LRPosRclRspStat] -> Switch3/1
  Constant12/1 -> Switch3/3
  Switch3/1 -> AND5/2
  [IfVeSMSeStNumConfig] -> Equal10/1
  Constant13/1 -> Equal10/2
  Equal10/1 -> Switch4/2
  [VeSignalLost2R_463_2L] -> Switch4/1
  Constant14/1 -> Switch4/3
  Switch4/1 -> AND3/2
  [SecRwRtStPosRclRspStat] -> Equal4/2
  Constant3/1 -> Equal11/2
  [IfVeSMSeStNumConfig] -> Equal11/1
  Equal11/1 -> Switch5/2
  Constant15/1 -> Switch5/3
  Equal5/1 -> Switch5/1
  Switch5/1 -> AND1/6
  Constant16/1 -> Equal12/2
  [IfVeSMSeStNumConfig] -> Equal12/1
  Equal12/1 -> Switch6/2
  [VeSignalLost2R_463_2L] -> Switch6/1
  Constant17/1 -> Switch6/3
  Switch6/1 -> AND7/1
  [SecRwRtStChldLkReq] -> Equal21/1
  [SecRwLtStChldLkReq] -> Equal27/1
  [SecRwLtStChldLkReq] -> Equal26/1
  Equal22/1 -> AND16/1
  Constant26/1 -> Equal21/2
  [SecRwRtStBkReclnUpwdDnwdPosOK] -> Equal20/1
  Constant19/1 -> Equal14/2
  [KeSMSwAcsMd32SecRwLtStBkReclnUpwdDnwdPos1] -> Equal17/2
  Constant27/1 -> Equal25/2
  AND18/1 -> [LugRtStChldLkOK], [RtStChldLkOK]
  AND11/1 -> AND13/1
  Equal13/1 -> AND10/2
  Constant22/1 -> Equal15/2
  Equal15/1 -> AND14/2
  Constant24/1 -> Equal22/2
  Constant23/1 -> Equal18/2
  Equal20/1 -> AND16/2
  Equal18/1 -> AND15/2
  AND13/1 -> AND12/1
  Equal19/1 -> AND15/1
  Constant25/1 -> Equal20/2
  SecRwRtStBkReclnUpwdDnwdPosV/1 -> Equal15/1
  Equal23/1 -> AND12/2
  Constant18/1 -> Equal27/2
  [KeSMSwAcsMd53SecRwRtStBkReclnUpwdDnwdPos1] -> Equal19/2
  Equal21/1 -> AND18/2
  Equal17/1 -> AND9/1
  AND16/1 -> AND18/1
  SecRwRtStBkReclnUpwdDnwdPos/1 -> Equal18/1, Equal19/1
  [SecRwRtStChldLkReq] -> Equal22/1
  Equal25/1 -> AND12/3
  Equal27/1 -> AND11/1
  AND12/1 -> [LugLtStChldLkOK]
  Equal26/1 -> AND13/2
  Constant21/1 -> Equal16/2
  Constant20/1 -> Equal13/2
  SecRwLtStBkReclnUpwdDnwdPosV/1 -> Equal13/1
  AND9/1 -> AND10/1
  AND10/1 -> [SecRwLtStBkReclnUpwdDnwdPosOK]
  [SecRwLtStBkReclnUpwdDnwdPosOK] -> Equal14/1
  Equal16/1 -> AND9/2
  AND15/1 -> AND14/1
  Constant28/1 -> Equal23/1, Equal26/2
  SecRwLtStBkReclnUpwdDnwdPos/1 -> Equal16/1, Equal17/1
  ThdRwLtStChldLkReq/1 -> Equal23/2
  [RtStChldLkOK] -> Equal25/1
  AND14/1 -> [SecRwRtStBkReclnUpwdDnwdPosOK]
  Equal14/1 -> AND11/2
  KeSMSuSecRwStBackPosDelta/1 -> [KeSMSuSecRwStBackPosDelta]
  Constant29/1 -> Equal28/2
  [LugLtStChldLkOK] -> Equal28/1
  [LugRtStChldLkOK] -> Equal29/1
  Constant30/1 -> Equal29/2
  Constant31/1 -> Equal30/2
  [IfVeSMSeStNumConfig] -> Equal30/1
  Constant32/1 -> Switch7/3
  Equal30/1 -> Switch7/2
  Equal28/1 -> Switch7/1
  Switch7/1 -> AND5/6
  Constant34/1 -> Switch8/3
  Equal31/1 -> Switch8/2
  Constant33/1 -> Equal31/2
  [IfVeSMSeStNumConfig] -> Equal31/1
  Equal29/1 -> Switch8/1
  Switch8/1 -> AND1/7
  SecRwLtStChldLkReq/1 -> [SecRwLtStChldLkReq]
  SecRwRtStChldLkReq/1 -> [SecRwRtStChldLkReq]
  VeSignalLost3R_46C_2L/1 -> AND7/2
  VeSignalLost3L_468_2L/1 -> AND3/1
  KeSMSwAcsMd32SecRwLtStBkReclnUpwdDnwdPos1/1 -> [KeSMSwAcsMd32SecRwLtStBkReclnUpwdDnwdPos1]
  KeSMSwAcsMd53SecRwRtStBkReclnUpwdDnwdPos1/1 -> [KeSMSwAcsMd53SecRwRtStBkReclnUpwdDnwdPos1]

== system PreCondition/PreConitionRunnable_sys/Subsystem3/CommCond / VehicleStatAndSpeed ==
  note: //E=N*0.015625
      | 0.0 - 511.984375 km/h
      | VehSpdAvgDrvn
  VehMovState : Inport
  VehSpdAvgDrvn : Inport  Port=2
  VehSpdAvgDrvnV : Inport  Port=3
  Constant : Constant  Value=VehMovState1.VehMvSts_Parked  OutDataTypeStr=Enum:VehMovState1
  Constant1 : Constant  Value=0  OutDataTypeStr=uint8
  Constant2 : Constant  Value=0  OutDataTypeStr=uint8
  Constant3 : Constant  Value=2  OutDataTypeStr=uint8
  Constant4 : Constant  OutDataTypeStr=uint8
  Data Type Conversion : DataTypeConversion  OutDataTypeStr=uint8
  Logical Operator : Logic  AllPortsSameDT=off  OutDataTypeStr=boolean
  Logical Operator1 : Logic  AllPortsSameDT=off  OutDataTypeStr=boolean
  Multiply : Gain  Gain=0.015625  OutDataTypeStr=fixdt(0,16,6)
  NOT1 : Logic  Operator=NOT  AllPortsSameDT=off  OutDataTypeStr=boolean
  NOT3 : Logic  Operator=NOT  AllPortsSameDT=off  OutDataTypeStr=boolean
  Relational Operator : RelationalOperator  Operator=<  OutDataTypeStr=boolean  RndMeth=Simplest
  Relational Operator1 : RelationalOperator  Operator===  OutDataTypeStr=boolean  RndMeth=Simplest
  Relational Operator2 : RelationalOperator  Operator===  OutDataTypeStr=boolean  RndMeth=Simplest
  Switch : Switch  Criteria=u2 > Threshold
  Switch1 : Switch  Criteria=u2 > Threshold
  vehSpeedModeAdjThrd : Constant  Value=2  OutDataTypeStr=fixdt(0,16,6)
  isVehStatAndSpeedOK : Outport  VectorParamsAs1DForOutWhenUnconnected=on
  DiagVehMovState : Outport  Port=2
  DiagVehSpdAvgDrvn : Outport  Port=3
  wires:
  Multiply/1 -> Relational Operator/1
  vehSpeedModeAdjThrd/1 -> Relational Operator/2
  Constant/1 -> Relational Operator1/2
  VehMovState/1 -> Relational Operator1/1
  Relational Operator/1 -> Switch1/2, Logical Operator1/1
  Relational Operator1/1 -> NOT3/1, Logical Operator/1
  Logical Operator/1 -> isVehStatAndSpeedOK/1
  Constant1/1 -> Relational Operator2/2
  Relational Operator2/1 -> NOT1/1, Logical Operator1/2
  Logical Operator1/1 -> Logical Operator/2
  VehSpdAvgDrvn/1 -> Multiply/1
  Constant3/1 -> Switch/1
  Switch/1 -> DiagVehSpdAvgDrvn/1
  NOT1/1 -> Switch/2
  Constant2/1 -> Switch1/1
  Constant4/1 -> Switch1/3
  Switch1/1 -> Switch/3
  VehSpdAvgDrvnV/1 -> Relational Operator2/1
  NOT3/1 -> Data Type Conversion/1
  Data Type Conversion/1 -> DiagVehMovState/1

== system PreCondition/PreConitionRunnable_sys/Subsystem3/CommCond /CommExitCond  ==
  VoltSts : Inport
  EnergyMgLdShdRq : Inport  Port=2
  PwrMd : Inport  Port=3
  AbgDly : Inport  Port=4
  isVehStatAndSpeedOK : Inport  Port=5
  AND : Logic  Operator=OR  Inputs=8  AllPortsSameDT=off  OutDataTypeStr=boolean
  Constant2 : Constant  Value=PowerMode1.PowerMode_Invalid
  Constant3 : Constant  Value=SeatSysVoltSt.CeSMS_SysVoltLow1
  Constant4 : Constant  Value=EnergyMgLdShdRq1.EnergyMgLdShdRq_LdShdLv3
  Constant5 : Constant  Value=SeatSysVoltSt.CeSMS_SysVoltLow2
  Constant6 : Constant  Value=SeatSysVoltSt.CeSMS_SysVoltHigh1
  Constant7 : Constant  Value=SeatSysVoltSt.CeSMS_SysVoltHigh2
  Equal{1..2,4..6} (5 alike) : RelationalOperator  Operator===  OutDataTypeStr=boolean  RndMeth=Simplest
  Equal3 : RelationalOperator  OutDataTypeStr=boolean  RndMeth=Simplest
  Logical Operator : Logic  Operator=NOT  AllPortsSameDT=off  OutDataTypeStr=boolean
  Logical Operator1 : Logic  Operator=NOT  AllPortsSameDT=off  OutDataTypeStr=boolean
  "CommExitCond " : Outport
  wires:
  Equal1/1 -> AND/1
  Constant2/1 -> Equal1/2
  Constant3/1 -> Equal2/2
  AND/1 -> "CommExitCond "/1
  EnergyMgLdShdRq/1 -> Equal3/1
  Constant4/1 -> Equal3/2
  [AbgDly] -> Logical Operator/1
  [isVehStatAndSpeedOK] -> Logical Operator1/1
  Constant5/1 -> Equal4/2
  VoltSts/1 -> Equal6/1, Equal5/1, Equal4/1, Equal2/1
  Constant6/1 -> Equal5/2
  Equal2/1 -> AND/2
  Equal4/1 -> AND/3
  Equal5/1 -> AND/4
  Constant7/1 -> Equal6/2
  Equal6/1 -> AND/5
  Equal3/1 -> AND/6
  Logical Operator/1 -> AND/7
  Logical Operator1/1 -> AND/8
  PwrMd/1 -> [PwrMd]
  [PwrMd] -> Equal1/1
  isVehStatAndSpeedOK/1 -> [isVehStatAndSpeedOK]
  AbgDly/1 -> [AbgDly]

== system PreCondition/PreConitionRunnable_sys/Subsystem3/CommCond /Subsystem ==
  note: $0=False; $1=True
  note: // 0是enable， 1是disable
  MmryRclImpctDisRq : Inport
  AbgDplyBckp : Inport  Port=2
  AbgDplyBckpV : Inport  Port=3
  VeSignalLostSDM_195_2L : Inport  Port=4
  VeSignalLostFireWall_1D2_2L : Inport  Port=5
  Constant : Constant  Value=0  OutDataTypeStr=uint8
  Constant1 : Constant  OutDataTypeStr=boolean
  Constant2 : Constant  Value=0  OutDataTypeStr=boolean
  Constant3 : Constant  Value=0  OutDataTypeStr=boolean
  Constant4 : Constant  Value=0  OutDataTypeStr=boolean
  Constant8 : Constant  Value=0  OutDataTypeStr=uint8
  Data Type Conversion : DataTypeConversion  OutDataTypeStr=uint8
  Equal : RelationalOperator  Operator===  OutDataTypeStr=boolean  RndMeth=Simplest
  NOT3 : Logic  Operator=NOT  AllPortsSameDT=off  OutDataTypeStr=boolean
  Relational Operator8 : RelationalOperator  Operator===  OutDataTypeStr=boolean  RndMeth=Simplest
  Switch{1..4} (4 alike) : Switch  Criteria=u2 > Threshold
  AbgDly : Outport
  wires:
  AbgDplyBckpV/1 -> Data Type Conversion/1
  Data Type Conversion/1 -> Relational Operator8/1
  Constant8/1 -> Relational Operator8/2
  Constant/1 -> Equal/2
  Equal/1 -> Switch1/2
  Constant1/1 -> Switch1/1
  Constant2/1 -> Switch1/3
  MmryRclImpctDisRq/1 -> Equal/1
  VeSignalLostSDM_195_2L/1 -> Switch2/2
  Switch1/1 -> Switch2/3
  Switch2/1 -> AbgDly/1
  VeSignalLostFireWall_1D2_2L/1 -> Switch3/2
  Switch4/1 -> Switch3/3
  Switch3/1 -> Switch2/1
  Constant3/1 -> Switch3/1
  Relational Operator8/1 -> Switch4/2
  Constant4/1 -> Switch4/3
  NOT3/1 -> Switch4/1
  AbgDplyBckp/1 -> NOT3/1

== system PreCondition/PreConitionRunnable_sys/Subsystem3/CommCond /VIPRcvyExitCond  ==
  VoltSts : Inport
  EnergyMgLdShdRq : Inport  Port=2
  PwrMd : Inport  Port=3
  AbgDly : Inport  Port=4
  VehMovState : Inport  Port=5
  AND : Logic  Operator=OR  Inputs=8  AllPortsSameDT=off  OutDataTypeStr=boolean
  Constant : Constant  Value=VehMovState1.VehMvSts_Invalid  OutDataTypeStr=Enum:VehMovState1
  Constant2 : Constant  Value=PowerMode1.PowerMode_Invalid
  Constant3 : Constant  Value=SeatSysVoltSt.CeSMS_SysVoltLow1
  Constant4 : Constant  Value=EnergyMgLdShdRq1.EnergyMgLdShdRq_LdShdLv3
  Constant5 : Constant  Value=SeatSysVoltSt.CeSMS_SysVoltLow2
  Constant6 : Constant  Value=SeatSysVoltSt.CeSMS_SysVoltHigh1
  Constant7 : Constant  Value=SeatSysVoltSt.CeSMS_SysVoltHigh2
  Equal{1..2,4..6} (5 alike) : RelationalOperator  Operator===  OutDataTypeStr=boolean  RndMeth=Simplest
  Equal3 : RelationalOperator  OutDataTypeStr=boolean  RndMeth=Simplest
  Logical Operator : Logic  Operator=NOT  AllPortsSameDT=off  OutDataTypeStr=boolean
  Relational Operator1 : RelationalOperator  Operator===  OutDataTypeStr=boolean  RndMeth=Simplest
  "CommExitCond " : Outport
  wires:
  Equal1/1 -> AND/1
  Constant2/1 -> Equal1/2
  Constant3/1 -> Equal2/2
  AND/1 -> "CommExitCond "/1
  EnergyMgLdShdRq/1 -> Equal3/1
  Constant4/1 -> Equal3/2
  [AbgDly] -> Logical Operator/1
  Constant5/1 -> Equal4/2
  VoltSts/1 -> Equal6/1, Equal5/1, Equal4/1, Equal2/1
  Constant6/1 -> Equal5/2
  Equal2/1 -> AND/2
  Equal4/1 -> AND/3
  Equal5/1 -> AND/4
  Constant7/1 -> Equal6/2
  Equal6/1 -> AND/5
  Equal3/1 -> AND/6
  Logical Operator/1 -> AND/7
  Relational Operator1/1 -> AND/8
  PwrMd/1 -> [PwrMd]
  [PwrMd] -> Equal1/1
  AbgDly/1 -> [AbgDly]
  VehMovState/1 -> Relational Operator1/1
  Constant/1 -> Relational Operator1/2
